simulink model "speedEstimatorPLL"  (R2024b)
settings: Solver=FixedStepAuto  StartTime=0.0  StopTime=Tend  FixedStep=Ts  RelTol=1e-3
values from neighbouring files (symbols this model uses):
  Ts = 1e-4    (= 0.0001)    [setup.m]    (also in test.m = 0.001)
undefined symbols (not defined in the file or in its folder): DiscIntNeverNeededParam, pll
settings Model: Creator=mhmok  LastModifiedBy=mhmok

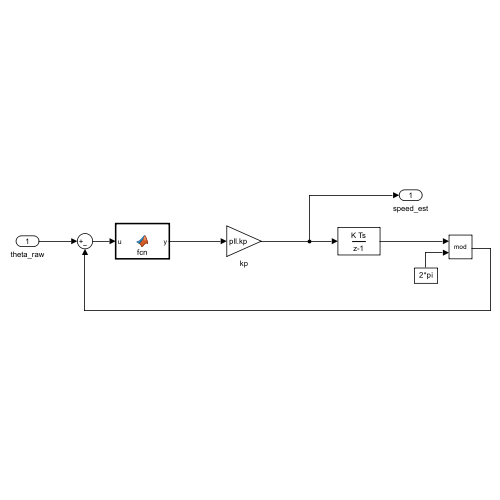
[thumbnail: Simulink's stored preview of the top-level diagram]
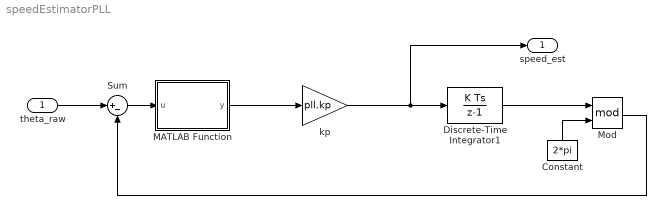
== system speedEstimatorPLL ==
  theta_raw : Inport
  Constant : Constant  Value=2*pi
  Discrete-Time Integrator1 : DiscreteIntegrator  gainval=1  SampleTime=Ts  ICPrevOutput=DiscIntNeverNeededParam  ICPrevScaledInput=DiscIntNeverNeededParam
  MATLAB Function : MATLAB Function  TreatAsAtomicUnit=on
  Mod : Math  Operator=mod
  Sum : Sum  Inputs=|+-
  kp : Gain  Gain=pll.kp
  speed_est : Outport
  wires:
  Sum/1 -> MATLAB Function/1(u)
  theta_raw/1 -> Sum/1
  Mod/1 -> Sum/2
  MATLAB Function/1(y) -> kp/1
  Constant/1 -> Mod/2
  Discrete-Time Integrator1/1 -> Mod/1
  kp/1 -> speed_est/1, Discrete-Time Integrator1/1

== matlab function speedEstimatorPLL/MATLAB Function ==
  data: u input; y output
function y = fcn(u)

y = u;

if y > pi
    y = y - 2*pi;
end

if y < -pi
    y = y + 2*pi;
end

end
